simulink library "dec2byte"  (Simulink 7.8)
settings: Solver=ode45  StartTime=0.0  StopTime=10.0  RelTol=1e-3
settings Model: Creator=KLJS168  LastModifiedBy=KLJS168

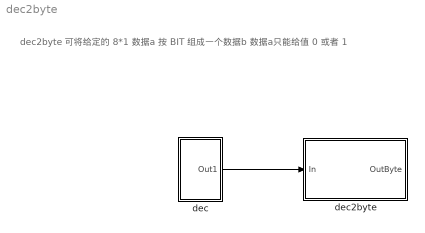
== system dec2byte ==
  note: dec2byte
      | 可将给定的 8*1 数据a 按 BIT 组成一个数据b
      | 数据a只能给值 0 或者 1
  dec : Subsystem
  dec2byte : Subsystem
  wires:
  dec/1(Out1) -> dec2byte/1(In)

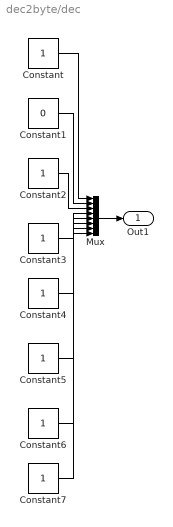
== system dec2byte/dec ==
  Constant{,2..7} (7 alike) : Constant
  Constant1 : Constant  Value=0
  Mux : Mux  Inputs=8
  Out1 : Outport
  wires:
  Constant/1 -> Mux/1
  Constant1/1 -> Mux/2
  Constant2/1 -> Mux/3
  Constant3/1 -> Mux/4
  Constant4/1 -> Mux/5
  Constant5/1 -> Mux/6
  Constant6/1 -> Mux/7
  Constant7/1 -> Mux/8
  Mux/1 -> Out1/1

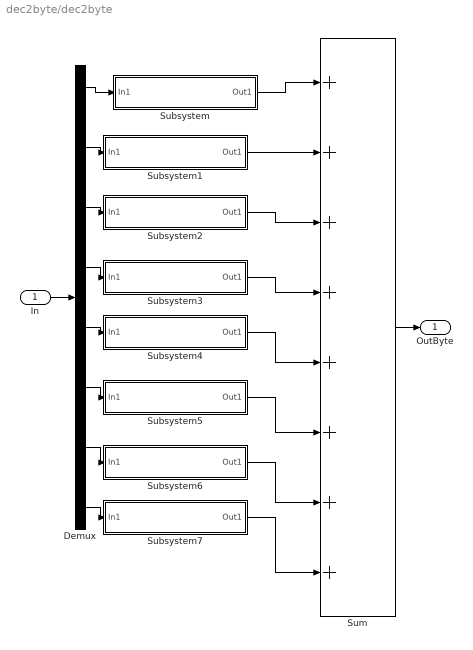
== system dec2byte/dec2byte ==
  In : Inport
  Demux : Demux  Outputs=8
  Subsystem : Subsystem  mask{power=0}
  Subsystem1 : Subsystem  mask{power=1}
  Subsystem2 : Subsystem  mask{power=2}
  Subsystem3 : Subsystem  mask{power=3}
  Subsystem4 : Subsystem  mask{power=4}
  Subsystem5 : Subsystem  mask{power=5}
  Subsystem6 : Subsystem  mask{power=6}
  Subsystem7 : Subsystem  mask{power=7}
  Sum : Sum  Inputs=++++++++
  OutByte : Outport
  wires:
  Demux/1 -> Subsystem/1(In1)
  Demux/2 -> Subsystem1/1(In1)
  Demux/3 -> Subsystem2/1(In1)
  Demux/4 -> Subsystem3/1(In1)
  Demux/5 -> Subsystem4/1(In1)
  Demux/6 -> Subsystem5/1(In1)
  Demux/7 -> Subsystem6/1(In1)
  Demux/8 -> Subsystem7/1(In1)
  Subsystem/1(Out1) -> Sum/1
  Subsystem1/1(Out1) -> Sum/2
  Subsystem2/1(Out1) -> Sum/3
  Subsystem3/1(Out1) -> Sum/4
  Subsystem4/1(Out1) -> Sum/5
  Subsystem5/1(Out1) -> Sum/6
  Subsystem6/1(Out1) -> Sum/7
  Subsystem7/1(Out1) -> Sum/8
  In/1 -> Demux/1
  Sum/1 -> OutByte/1

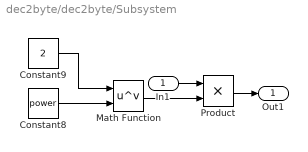
== system dec2byte/dec2byte/Subsystem ==
  In1 : Inport
  Constant8 : Constant  Value=power
  Constant9 : Constant  Value=2
  Math Function : Math  Operator=pow  SaturateOnIntegerOverflow=on
  Product : Product  RndMeth=Zero
  Out1 : Outport
  wires:
  Constant8/1 -> Math Function/2
  Constant9/1 -> Math Function/1
  Math Function/1 -> Product/2
  In1/1 -> Product/1
  Product/1 -> Out1/1

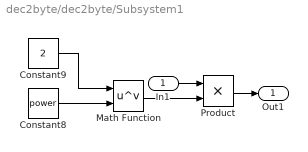
== system dec2byte/dec2byte/Subsystem1 ==
  In1 : Inport
  Constant8 : Constant  Value=power
  Constant9 : Constant  Value=2
  Math Function : Math  Operator=pow  SaturateOnIntegerOverflow=on
  Product : Product  RndMeth=Zero
  Out1 : Outport
  wires:
  Product/1 -> Out1/1
  In1/1 -> Product/1
  Math Function/1 -> Product/2
  Constant9/1 -> Math Function/1
  Constant8/1 -> Math Function/2

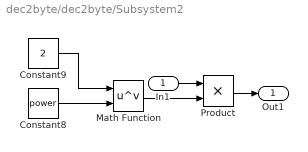
== system dec2byte/dec2byte/Subsystem2 ==
  In1 : Inport
  Constant8 : Constant  Value=power
  Constant9 : Constant  Value=2
  Math Function : Math  Operator=pow  SaturateOnIntegerOverflow=on
  Product : Product  RndMeth=Zero
  Out1 : Outport
  wires:
  Constant8/1 -> Math Function/2
  Constant9/1 -> Math Function/1
  Math Function/1 -> Product/2
  In1/1 -> Product/1
  Product/1 -> Out1/1

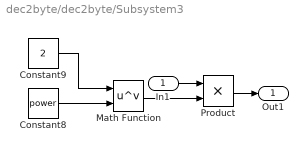
== system dec2byte/dec2byte/Subsystem3 ==
  In1 : Inport
  Constant8 : Constant  Value=power
  Constant9 : Constant  Value=2
  Math Function : Math  Operator=pow  SaturateOnIntegerOverflow=on
  Product : Product  RndMeth=Zero
  Out1 : Outport
  wires:
  Product/1 -> Out1/1
  In1/1 -> Product/1
  Math Function/1 -> Product/2
  Constant9/1 -> Math Function/1
  Constant8/1 -> Math Function/2

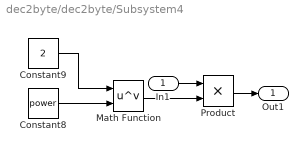
== system dec2byte/dec2byte/Subsystem4 ==
  In1 : Inport
  Constant8 : Constant  Value=power
  Constant9 : Constant  Value=2
  Math Function : Math  Operator=pow  SaturateOnIntegerOverflow=on
  Product : Product  RndMeth=Zero
  Out1 : Outport
  wires:
  Constant8/1 -> Math Function/2
  Constant9/1 -> Math Function/1
  Math Function/1 -> Product/2
  In1/1 -> Product/1
  Product/1 -> Out1/1

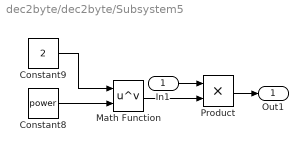
== system dec2byte/dec2byte/Subsystem5 ==
  In1 : Inport
  Constant8 : Constant  Value=power
  Constant9 : Constant  Value=2
  Math Function : Math  Operator=pow  SaturateOnIntegerOverflow=on
  Product : Product  RndMeth=Zero
  Out1 : Outport
  wires:
  Product/1 -> Out1/1
  In1/1 -> Product/1
  Math Function/1 -> Product/2
  Constant9/1 -> Math Function/1
  Constant8/1 -> Math Function/2

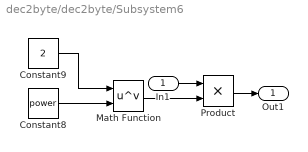
== system dec2byte/dec2byte/Subsystem6 ==
  In1 : Inport
  Constant8 : Constant  Value=power
  Constant9 : Constant  Value=2
  Math Function : Math  Operator=pow  SaturateOnIntegerOverflow=on
  Product : Product  RndMeth=Zero
  Out1 : Outport
  wires:
  Constant8/1 -> Math Function/2
  Constant9/1 -> Math Function/1
  Math Function/1 -> Product/2
  In1/1 -> Product/1
  Product/1 -> Out1/1

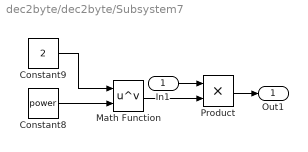
== system dec2byte/dec2byte/Subsystem7 ==
  In1 : Inport
  Constant8 : Constant  Value=power
  Constant9 : Constant  Value=2
  Math Function : Math  Operator=pow  SaturateOnIntegerOverflow=on
  Product : Product  RndMeth=Zero
  Out1 : Outport
  wires:
  Product/1 -> Out1/1
  In1/1 -> Product/1
  Math Function/1 -> Product/2
  Constant9/1 -> Math Function/1
  Constant8/1 -> Math Function/2
